simulink model "PUMA_PID_dis"  (Simulink 8.9)
settings: Solver=ode15s  StartTime=0  StopTime=5  MaxStep=0.02  RelTol=1e-3  EnableMultiTasking=on
undefined symbols (not defined in the file): sfunxyz
libraries: aerolibutil x17, simulink x7
(part 1 of 3)
settings Model: Creator=LAAAS3  LastModifiedBy=bmoh1
settings OptimizationCC: InitFltsAndDblsToZero=on
settings DebuggingCC: SaveWithParameterizedLinksMsg=none  SignalResolutionControl=TryResolveAllWithWarning  MaxConsecutiveZCsMsg=none  SolverPrmCheckMsg=warning  MultiTaskDSMMsg=warning  MultiTaskCondExecSysMsg=none  FcnCallInpInsideContextMsg=error  StateNameClashWarn=none
settings GRTTargetCC: TargetFcnLib=ansi_tfl_tmw.mat  GeneratePreprocessorConditionals=Use local settings

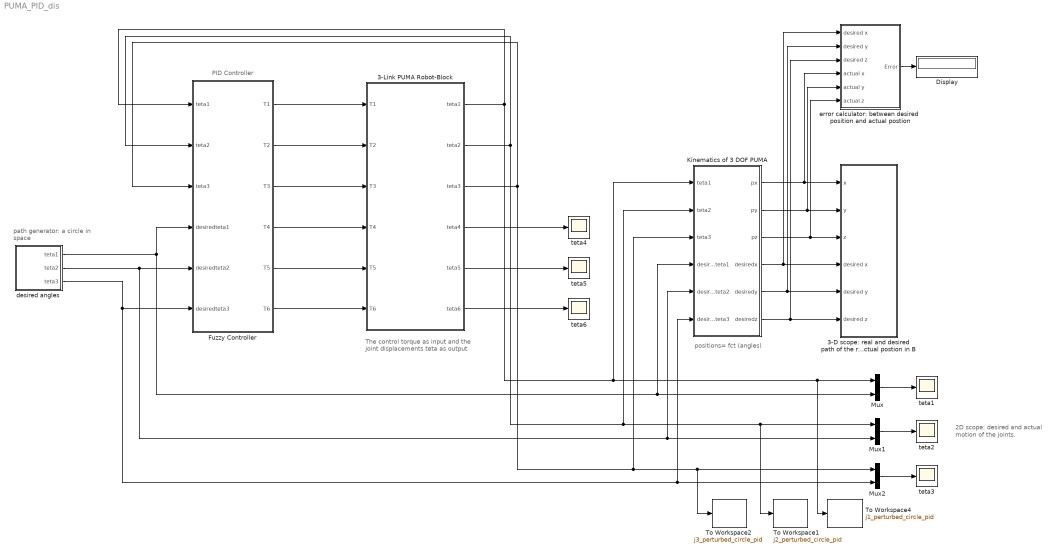
== system PUMA_PID_dis ==
  note: PID Controller
  note: 2D scope: desired and actual
      |          motion of the joints.
  note: The control torque as input and the
      | joint displacements teta as output
  note: path generator: a
      | circle in space
  note: positions= fct (angles)
  "3-D scope: real and desired path of the robot  desired position in G and actual postion in B " : Subsystem
  "3-Link PUMA Robot-Block " : Subsystem  mask{UIm1=0, UIm2=0, UIm3=0, UIm4=0, UIm5=0, UIm6=0, UI1=0, UI2=0, UI3=0, UI4=0, UI5=0, UI6=0, UI7=0, UI8=0, UI9=0, UI10=0, UI11=0, UI12=0, UI13=0, UI14=0, UI15=0, UI16=0, UI17=0, UI18=0, UI19=0, UI20=0, UI21=0, UI22=0, UI23=0, UG1=0, UG2=0, UG3=0, UG4=0, UG5=0}
      mask prompts: UIm1 "UIm1 +-0.27"; UIm2 "UIm2 +-0.54"; UIm3 "UIm3 +-0.093"; UIm4 "UIm4 +-0.016"; UIm5 "UIm5 +-0.014"; UIm6 "UIm6 +-0.016"; UI1 "UI1 +-0.05"; UI2 "UI2 +-0.07"; UI3 "UI3 +-0.05"; UI4 "UI4 +-0.02"; UI5 "UI5 +-0.031"; UI6 "UI6 +-0.016"; UI7 "UI7 +-0.029"; UI8 "UI8 +-0.014"; UI9 "UI9 +-0.012"; UI10 "UI10 +-0.0022"; UI11 "UI11 +-0.007"; UI12 "UI12 +-0.0011"; UI13 "UI13 +-0.0009"; UI14 "UI14 +-0.00007"; UI15 "UI15 +-0.0003"; UI16 "UI16 +-0.0003"; UI17 "UI17 +-0.0003"; UI18 "UI18 +-0.00013"; UI19 "UI19 +-0.0014"; UI20 "UI20 +-0.0008"; UI21 "UI21 +-0.0006"; UI22 "UI22 +-0.000015"; UI23 "UI23 +-0.00002"; UG1 "UG1 +-0.5"; UG2 "UG2 +-0.2"; UG3 "UG3 +-0.5"; UG4 "UG4 +-0.025"; UG5 "UG5 +-0.0056"
  Display : Display
  Fuzzy Controller : Subsystem
  Kinematics of 3 DOF PUMA : MATLAB Function  TreatAsAtomicUnit=on
  Mux : Mux  Inputs=2
  Mux1 : Mux  Inputs=2
  Mux2 : Mux  Inputs=2
  To Workspace1 : ToWorkspace  VariableName=j2_perturbed_circle_pid  SaveFormat=Timeseries  SampleTime=-1
      settings: Save2DSignal=2-D array (concatenate along first dimension)
  To Workspace2 : ToWorkspace  VariableName=j3_perturbed_circle_pid  SaveFormat=Timeseries  SampleTime=-1
      settings: Save2DSignal=2-D array (concatenate along first dimension)
  To Workspace4 : ToWorkspace  VariableName=j1_perturbed_circle_pid  SaveFormat=Timeseries  SampleTime=-1
      settings: Save2DSignal=2-D array (concatenate along first dimension)
  "desired angles  " : Subsystem
  error calculator: between desired  position and actual postion : Subsystem
  teta{1..6} (6 alike) : Scope
  wires:
  "3-Link PUMA Robot-Block "/3(teta3) -> To Workspace2/1, Mux2/1, Kinematics of 3 DOF PUMA/3(teta3), Fuzzy Controller/3(teta3)
  "3-Link PUMA Robot-Block "/4(teta4) -> teta4/1
  "3-Link PUMA Robot-Block "/5(teta5) -> teta5/1
  "3-Link PUMA Robot-Block "/6(teta6) -> teta6/1
  "desired angles  "/1(teta1) -> Mux/2, Kinematics of 3 DOF PUMA/4(desiredteta1), Fuzzy Controller/4(desiredteta1)
  "desired angles  "/2(teta2) -> Mux1/2, Kinematics of 3 DOF PUMA/5(desiredteta2), Fuzzy Controller/5(desiredteta2)
  "desired angles  "/3(teta3) -> Mux2/2, Kinematics of 3 DOF PUMA/6(desiredteta3), Fuzzy Controller/6(desiredteta3)
  error calculator: between desired  position and actual postion/1(Error) -> Display/1
  Kinematics of 3 DOF PUMA/1(px) -> "3-D scope: real and desired path of the robot  desired position in G and actual postion in B "/1(x), error calculator: between desired  position and actual postion/4(actual x)
  Kinematics of 3 DOF PUMA/2(py) -> "3-D scope: real and desired path of the robot  desired position in G and actual postion in B "/2(y), error calculator: between desired  position and actual postion/5(actual y)
  Kinematics of 3 DOF PUMA/3(pz) -> "3-D scope: real and desired path of the robot  desired position in G and actual postion in B "/3(z), error calculator: between desired  position and actual postion/6(actual z)
  Kinematics of 3 DOF PUMA/4(desiredx) -> "3-D scope: real and desired path of the robot  desired position in G and actual postion in B "/4(desired x), error calculator: between desired  position and actual postion/1(desired x)
  Kinematics of 3 DOF PUMA/5(desiredy) -> "3-D scope: real and desired path of the robot  desired position in G and actual postion in B "/5(desired y), error calculator: between desired  position and actual postion/2(desired y)
  Kinematics of 3 DOF PUMA/6(desiredz) -> "3-D scope: real and desired path of the robot  desired position in G and actual postion in B "/6(desired z), error calculator: between desired  position and actual postion/3(desired z)
  Mux/1 -> teta1/1
  Mux1/1 -> teta2/1
  Mux2/1 -> teta3/1
  Fuzzy Controller/4(T4) -> "3-Link PUMA Robot-Block "/4(T4)
  Fuzzy Controller/5(T5) -> "3-Link PUMA Robot-Block "/5(T5)
  Fuzzy Controller/6(T6) -> "3-Link PUMA Robot-Block "/6(T6)
  Fuzzy Controller/1(T1) -> "3-Link PUMA Robot-Block "/1(T1)
  Fuzzy Controller/2(T2) -> "3-Link PUMA Robot-Block "/2(T2)
  Fuzzy Controller/3(T3) -> "3-Link PUMA Robot-Block "/3(T3)
  "3-Link PUMA Robot-Block "/2(teta2) -> To Workspace1/1, Mux1/1, Kinematics of 3 DOF PUMA/2(teta2), Fuzzy Controller/2(teta2)
  "3-Link PUMA Robot-Block "/1(teta1) -> To Workspace4/1, Mux/1, Kinematics of 3 DOF PUMA/1(teta1), Fuzzy Controller/1(teta1)

== system PUMA_PID_dis/3-D scope: real and desired path of the robot  desired position in G and actual postion in B  ==
  x : Inport
  y : Inport  Port=2
  z : Inport  Port=3
  desired x : Inport  Port=4
  desired y : Inport  Port=5
  desired z : Inport  Port=6
  Demux : Demux  Outputs=[2 2 2]
  Mux : Mux  Inputs=3
  Mux1 : Mux  Inputs=3
  Mux3 : Mux  Inputs=2
  To Workspace1 : ToWorkspace  VariableName=xyz_pert_circle_pid  SaveFormat=Timeseries  SampleTime=-1
      settings: Save2DSignal=2-D array (concatenate along first dimension)
  Transpose : Selector  InputPortWidth=3*2  IndexOptions=Index vector (dialog)  Indices=reshape(reshape(1:3*2,3,2)',3*2,1)  OutputSizes=1
  XYZ Graph : Subsystem  LoadFcn=sfunxyz([],[],[],'LoadBlock')  StartFcn=sfunxyz([],[],[],'Start')  StopFcn=sfunxyz([],[],[],'Stop')  mask(XYZ multiscope){np=2, xlim=[-1 1], ylim=[-1 1], zlim=[-1 1], cp=[3 2 1], gd=on, st=0.1}
      mask prompts: np "Number of lines"; xlim "[xmin xmax]"; ylim "[ymin ymax]"; zlim "[zmin zmax]"; cp "Camera position (use [0 0 1] for 2D XY view)"; gd "Grid"; st "Sample time:"
      mask help:
      | Multidimensional XYZ scope using MATLAB graph window.
      |    X,Y,Z coordinates are respectively the first,second, and third input.
      |    Enter the number of lines, the XYZ ranges, the camera position,
      |    and the sampling time, as mask parameters.
      settings: CopyFcn=sfunxyz([],[],[],'CopyBlock')  DeleteFcn=sfunxyz([],[],[],'DeleteBlock')  NameChangeFcn=sfunxyz([],[],[],'NameChange')
      mask Help:
      | This block can be used to explore limit cycles.
      |    Look at the m-file sfunxyz.m to see how it works.
      mask Display: plot([.05 .95 .95 .05 .05],[.45 .45 .95 .95 .45], 0.5+cos(0:0.1:2*pi)*0.3,0.7+sin(0:0.1:2*pi)*0.2)
  wires:
  Mux1/1 -> Mux3/2  "Line2 XYZ"
  Mux3/1 -> Transpose/1
  Transpose/1 -> Demux/1
  Demux/1 -> XYZ Graph/1(x)  "X Coordinates"
  Demux/2 -> XYZ Graph/2(y)  "Y Coordinates"
  Demux/3 -> XYZ Graph/3(z)  "Z Coordinates"
  x/1 -> Mux/1
  y/1 -> Mux/2
  z/1 -> Mux/3
  Mux/1 -> To Workspace1/1, Mux3/1  "Line1 XYZ"
  desired x/1 -> Mux1/1
  desired y/1 -> Mux1/2
  desired z/1 -> Mux1/3

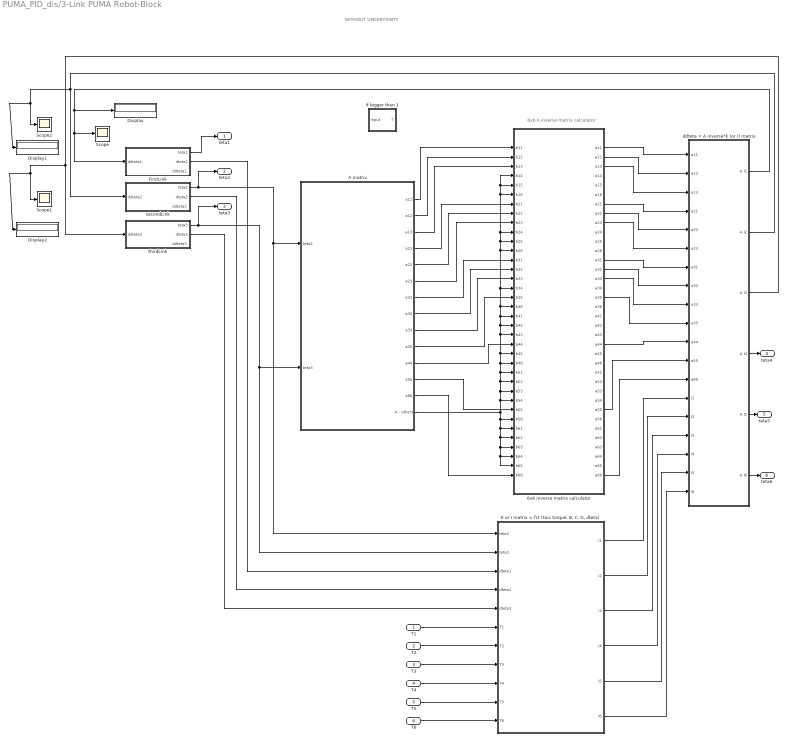
== system PUMA_PID_dis/3-Link PUMA Robot-Block  ==
  note: 6x6 A inverse matrix calculator
  note: WITHOUT UNCERTAINTY
  T1 : Inport
  T2 : Inport  Port=2
  T3 : Inport  Port=3
  T4 : Inport  Port=4
  T5 : Inport  Port=5
  T6 : Inport  Port=6
  6x6 inverse matrix calculator : MATLAB Function  TreatAsAtomicUnit=on
  A matrix : Subsystem
  Display : Display
  Display1 : Display
  Display2 : Display
  FirstLink : Subsystem  mask(FirstLink){}
      mask help:
      | the first link of the robot. the input is the double derivative of teta1, the displacement of
      | the link.
      | the outputs are: teta1 the displacement of the first joint, dteta1 the velocity of the
      | first joint.
      | NOTE: the link is connected to a revolute joint.
      mask Help:
      | the first link of the robot. the input is the double derivative of teta1, the displacement of
      | the link.
      | the outputs are: teta1 the displacement of the first joint, dteta1 the velocity of the
      | first joint.
      | NOTE: the link is connected to a revolute joint.
  "K or I matrix = fct (tau: torque, B, C, G, dteta) " : Subsystem
  Scope : Scope
  Scope1 : Scope
  Scope2 : Scope
  "ddteta = A inverse*k (or I) matrix " : Subsystem
  if bigger than 1 : MATLAB Function  TreatAsAtomicUnit=on
  secondLink : Subsystem  mask(SecondLink){}
      mask help:
      | the first link of the robot. the input is the double derivative of teta1, the displacement of
      | the link.
      | the outputs are: teta1 the displacement of the second joint, dteta1 the velocity of the
      | second joint.
      | NOTE: the link is connected to a revolute joint.
      mask Help:
      | the secod link of the robot. the input is the double derivative of teta2, the displacement of
      | the link.
      | the outputs are: teta2 the displacement of the second joint, dteta2 the velocity of the
      | second joint.
      | NOTE: the link is connected to a revolute joint.
  thirdLink : Subsystem  mask(ThirdLink){}
      mask help:
      | the third link of the robot. the input is the double derivative of teta3, the displacement of
      | the link.
      | the outputs are: teta3 the displacement of the third joint, dteta3 the velocity of the
      | third joint.
      | NOTE: the link is connected to a revolute joint.
      mask Help:
      | the third link of the robot. the input is the double derivative of teta3, the displacement of
      | the link.
      | the outputs are: teta3 the displacement of the third joint, dteta3 the velocity of the
      | third joint.
      | NOTE: the link is connected to a revolute joint.
  teta1 : Outport
  teta2 : Outport  Port=2
  teta3 : Outport  Port=3
  teta4 : Outport  Port=4
  teta5 : Outport  Port=5
  teta6 : Outport  Port=6
  wires:
  A matrix/1(a11) -> 6x6 inverse matrix calculator/1(b11)
  A matrix/2(a12) -> 6x6 inverse matrix calculator/2(b12)
  A matrix/3(a13) -> 6x6 inverse matrix calculator/3(b13)
  A matrix/4(a21) -> 6x6 inverse matrix calculator/7(b21)
  A matrix/5(a22) -> 6x6 inverse matrix calculator/8(b22)
  A matrix/6(a23) -> 6x6 inverse matrix calculator/9(b23)
  A matrix/7(a31) -> 6x6 inverse matrix calculator/13(b31)
  A matrix/8(a32) -> 6x6 inverse matrix calculator/14(b32)
  A matrix/9(a33) -> 6x6 inverse matrix calculator/15(b33)
  A matrix/10(a35) -> 6x6 inverse matrix calculator/17(b35)
  A matrix/11(a44) -> 6x6 inverse matrix calculator/22(b44)
  A matrix/12(a55) -> 6x6 inverse matrix calculator/29(b55)
  A matrix/13(a66) -> 6x6 inverse matrix calculator/36(b66)
  A matrix/14(A - others) -> 6x6 inverse matrix calculator/30(b56), 6x6 inverse matrix calculator/35(b65), 6x6 inverse matrix calculator/34(b64), 6x6 inverse matrix calculator/33(b63), 6x6 inverse matrix calculator/32(b62), 6x6 inverse matrix calculator/31(b61), 6x6 inverse matrix calculator/28(b54), 6x6 inverse matrix calculator/27(b53), 6x6 inverse matrix calculator/26(b52), 6x6 inverse matrix calculator/25(b51), 6x6 inverse matrix calculator/24(b46), 6x6 inverse matrix calculator/23(b45), 6x6 inverse matrix calculator/21(b43), 6x6 inverse matrix calculator/20(b42), 6x6 inverse matrix calculator/19(b41), 6x6 inverse matrix calculator/18(b36), 6x6 inverse matrix calculator/16(b34), 6x6 inverse matrix calculator/12(b26), 6x6 inverse matrix calculator/11(b25), 6x6 inverse matrix calculator/10(b24), 6x6 inverse matrix calculator/6(b16), 6x6 inverse matrix calculator/4(b14), 6x6 inverse matrix calculator/5(b15)
  secondLink/1(teta2) -> "K or I matrix = fct (tau: torque, B, C, G, dteta) "/1(teta2), A matrix/1(teta2), teta2/1
  thirdLink/1(teta3) -> teta3/1, "K or I matrix = fct (tau: torque, B, C, G, dteta) "/2(teta3), A matrix/2(teta3)
  FirstLink/2(dteta1) -> "K or I matrix = fct (tau: torque, B, C, G, dteta) "/3(dteta1)
  secondLink/2(dteta2) -> "K or I matrix = fct (tau: torque, B, C, G, dteta) "/4(dteta2)
  thirdLink/2(dteta3) -> "K or I matrix = fct (tau: torque, B, C, G, dteta) "/5(dteta3)
  T1/1 -> "K or I matrix = fct (tau: torque, B, C, G, dteta) "/6(T1)
  T2/1 -> "K or I matrix = fct (tau: torque, B, C, G, dteta) "/7(T2)
  T3/1 -> "K or I matrix = fct (tau: torque, B, C, G, dteta) "/8(T3)
  T4/1 -> "K or I matrix = fct (tau: torque, B, C, G, dteta) "/9(T4)
  T5/1 -> "K or I matrix = fct (tau: torque, B, C, G, dteta) "/10(T5)
  T6/1 -> "K or I matrix = fct (tau: torque, B, C, G, dteta) "/11(T6)
  "ddteta = A inverse*k (or I) matrix "/1(A.I1) -> Display/1, Scope/1, FirstLink/1(ddteta1)
  FirstLink/1(teta1) -> teta1/1
  "ddteta = A inverse*k (or I) matrix "/4(A.I4) -> teta4/1
  "ddteta = A inverse*k (or I) matrix "/5(A.I5) -> teta5/1
  "ddteta = A inverse*k (or I) matrix "/6(A.I6) -> teta6/1
  "K or I matrix = fct (tau: torque, B, C, G, dteta) "/1(I1) -> "ddteta = A inverse*k (or I) matrix "/14(I1)
  "K or I matrix = fct (tau: torque, B, C, G, dteta) "/2(I2) -> "ddteta = A inverse*k (or I) matrix "/15(I2)
  "K or I matrix = fct (tau: torque, B, C, G, dteta) "/3(I3) -> "ddteta = A inverse*k (or I) matrix "/16(I3)
  6x6 inverse matrix calculator/1(a11) -> "ddteta = A inverse*k (or I) matrix "/1(a11)
  6x6 inverse matrix calculator/2(a12) -> "ddteta = A inverse*k (or I) matrix "/2(a12)
  6x6 inverse matrix calculator/3(a13) -> "ddteta = A inverse*k (or I) matrix "/3(a13)
  6x6 inverse matrix calculator/7(a21) -> "ddteta = A inverse*k (or I) matrix "/4(a21)
  6x6 inverse matrix calculator/8(a22) -> "ddteta = A inverse*k (or I) matrix "/5(a22)
  6x6 inverse matrix calculator/9(a23) -> "ddteta = A inverse*k (or I) matrix "/6(a23)
  6x6 inverse matrix calculator/13(a31) -> "ddteta = A inverse*k (or I) matrix "/7(a31)
  6x6 inverse matrix calculator/14(a32) -> "ddteta = A inverse*k (or I) matrix "/8(a32)
  6x6 inverse matrix calculator/15(a33) -> "ddteta = A inverse*k (or I) matrix "/9(a33)
  6x6 inverse matrix calculator/17(a35) -> "ddteta = A inverse*k (or I) matrix "/10(a35)
  6x6 inverse matrix calculator/22(a44) -> "ddteta = A inverse*k (or I) matrix "/11(a44)
  6x6 inverse matrix calculator/29(a55) -> "ddteta = A inverse*k (or I) matrix "/12(a55)
  6x6 inverse matrix calculator/36(a66) -> "ddteta = A inverse*k (or I) matrix "/13(a66)
  "K or I matrix = fct (tau: torque, B, C, G, dteta) "/4(I4) -> "ddteta = A inverse*k (or I) matrix "/17(I4)
  "K or I matrix = fct (tau: torque, B, C, G, dteta) "/5(I5) -> "ddteta = A inverse*k (or I) matrix "/18(I5)
  "K or I matrix = fct (tau: torque, B, C, G, dteta) "/6(I6) -> "ddteta = A inverse*k (or I) matrix "/19(I6)
  "ddteta = A inverse*k (or I) matrix "/3(A.I3) -> Display2/1, Scope1/1, thirdLink/1(ddteta3)
  "ddteta = A inverse*k (or I) matrix "/2(A.I2) -> Display1/1, Scope2/1, secondLink/1(ddteta2)

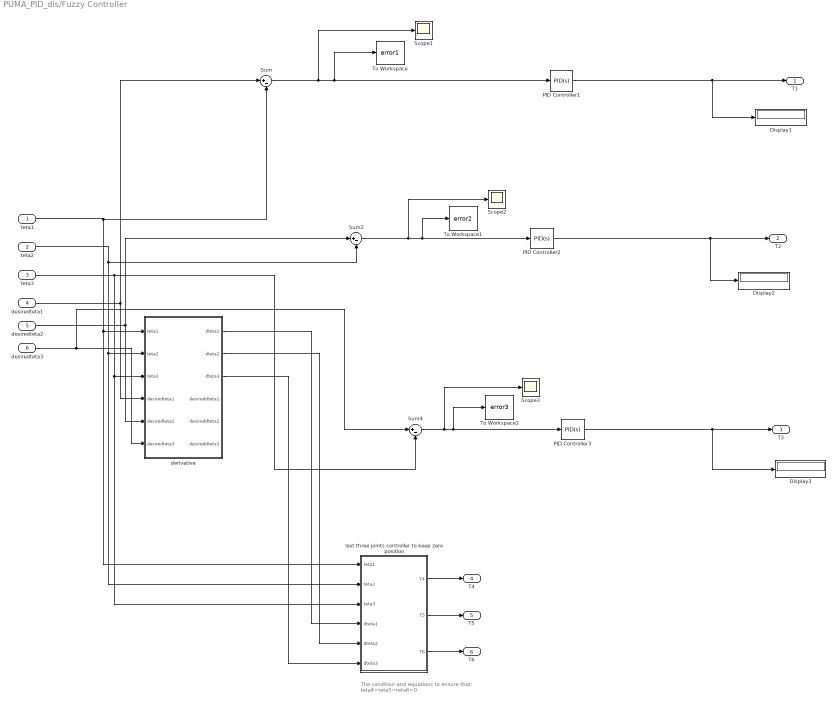
== system PUMA_PID_dis/Fuzzy Controller ==
  note: The condition and equations to ensure that:
      |                    teta4=teta5=teta6=0
  teta1 : Inport
  teta2 : Inport  Port=2
  teta3 : Inport  Port=3
  desiredteta1 : Inport  Port=4
  desiredteta2 : Inport  Port=5
  desiredteta3 : Inport  Port=6
  Display1 : Display
  Display2 : Display
  Display3 : Display
  PID Controller1 : simulink/Continuous/PID Controller  Controller=PID  TimeDomain=Continuous-time  SampleTime=-1  IntegratorMethod=Forward Euler  FilterMethod=Forward Euler  Form=Parallel  UseFilter=on  ControllerParametersSource=internal  P=100  I=1  D=60  N=38.4128689358779  InitialConditionSource=internal  InitialConditionForIntegrator=0  InitialConditionForFilter=0  ExternalReset=none  LimitOutput=off  UpperSaturationLimit=inf  LowerSaturationLimit=-inf  LinearizeAsGain=on  AntiWindupMode=none  Kb=1  TrackingMode=off  Kt=1  PParamMin=[]  PParamMax=[]  IParamMin=[]  IParamMax=[]  DParamMin=[]  DParamMax=[]  NParamMin=[]  NParamMax=[]  KbParamMin=[]  KbParamMax=[]  KtParamMin=[]  KtParamMax=[]  POutMin=[]  POutMax=[]  IOutMin=[]  IOutMax=[]  DOutMin=[]  DOutMax=[]  NOutMin=[]  NOutMax=[]  KbOutMin=[]  KbOutMax=[]  KtOutMin=[]  KtOutMax=[]  IntegratorOutMin=[]  IntegratorOutMax=[]  FilterOutMin=[]  FilterOutMax=[]  SumOutMin=[]  SumOutMax=[]  SumI1OutMin=[]  SumI1OutMax=[]  SumI2OutMin=[]  SumI2OutMax=[]  SumI3OutMin=[]  SumI3OutMax=[]  SumDOutMin=[]  SumDOutMax=[]  SaturationOutMin=[]  SaturationOutMax=[]  IntegratorContinuousStateAttributes=''  IntegratorStateMustResolveToSignalObject=off  IntegratorRTWStateStorageClass=Auto  FilterContinuousStateAttributes=''  FilterStateMustResolveToSignalObject=off  FilterRTWStateStorageClass=Auto  DifferentiatorICPrevScaledInput=0  DifferentiatorOutMin=[]  DifferentiatorOutMax=[]  InitialConditionSetting=State (most efficient)
  PID Controller2 : simulink/Continuous/PID Controller  Controller=PID  TimeDomain=Continuous-time  SampleTime=-1  IntegratorMethod=Forward Euler  FilterMethod=Forward Euler  Form=Parallel  UseFilter=on  ControllerParametersSource=internal  P=259.447618274315  I=64.6556993070995  D=70.4723983176902  N=17.7020176521094  InitialConditionSource=internal  InitialConditionForIntegrator=0  InitialConditionForFilter=0  ExternalReset=none  LimitOutput=off  UpperSaturationLimit=inf  LowerSaturationLimit=-inf  LinearizeAsGain=on  AntiWindupMode=none  Kb=1  TrackingMode=off  Kt=1  PParamMin=[]  PParamMax=[]  IParamMin=[]  IParamMax=[]  DParamMin=[]  DParamMax=[]  NParamMin=[]  NParamMax=[]  KbParamMin=[]  KbParamMax=[]  KtParamMin=[]  KtParamMax=[]  POutMin=[]  POutMax=[]  IOutMin=[]  IOutMax=[]  DOutMin=[]  DOutMax=[]  NOutMin=[]  NOutMax=[]  KbOutMin=[]  KbOutMax=[]  KtOutMin=[]  KtOutMax=[]  IntegratorOutMin=[]  IntegratorOutMax=[]  FilterOutMin=[]  FilterOutMax=[]  SumOutMin=[]  SumOutMax=[]  SumI1OutMin=[]  SumI1OutMax=[]  SumI2OutMin=[]  SumI2OutMax=[]  SumI3OutMin=[]  SumI3OutMax=[]  SumDOutMin=[]  SumDOutMax=[]  SaturationOutMin=[]  SaturationOutMax=[]  IntegratorContinuousStateAttributes=''  IntegratorStateMustResolveToSignalObject=off  IntegratorRTWStateStorageClass=Auto  FilterContinuousStateAttributes=''  FilterStateMustResolveToSignalObject=off  FilterRTWStateStorageClass=Auto  DifferentiatorICPrevScaledInput=0  DifferentiatorOutMin=[]  DifferentiatorOutMax=[]  InitialConditionSetting=State (most efficient)
  PID Controller3 : simulink/Continuous/PID Controller  Controller=PID  TimeDomain=Continuous-time  SampleTime=-1  IntegratorMethod=Forward Euler  FilterMethod=Forward Euler  Form=Parallel  UseFilter=on  ControllerParametersSource=internal  P=298.294353009705  I=370.312527265234  D=35  N=2913.028427628  InitialConditionSource=internal  InitialConditionForIntegrator=0  InitialConditionForFilter=0  ExternalReset=none  LimitOutput=off  UpperSaturationLimit=inf  LowerSaturationLimit=-inf  LinearizeAsGain=on  AntiWindupMode=none  Kb=1  TrackingMode=off  Kt=1  PParamMin=[]  PParamMax=[]  IParamMin=[]  IParamMax=[]  DParamMin=[]  DParamMax=[]  NParamMin=[]  NParamMax=[]  KbParamMin=[]  KbParamMax=[]  KtParamMin=[]  KtParamMax=[]  POutMin=[]  POutMax=[]  IOutMin=[]  IOutMax=[]  DOutMin=[]  DOutMax=[]  NOutMin=[]  NOutMax=[]  KbOutMin=[]  KbOutMax=[]  KtOutMin=[]  KtOutMax=[]  IntegratorOutMin=[]  IntegratorOutMax=[]  FilterOutMin=[]  FilterOutMax=[]  SumOutMin=[]  SumOutMax=[]  SumI1OutMin=[]  SumI1OutMax=[]  SumI2OutMin=[]  SumI2OutMax=[]  SumI3OutMin=[]  SumI3OutMax=[]  SumDOutMin=[]  SumDOutMax=[]  SaturationOutMin=[]  SaturationOutMax=[]  IntegratorContinuousStateAttributes=''  IntegratorStateMustResolveToSignalObject=off  IntegratorRTWStateStorageClass=Auto  FilterContinuousStateAttributes=''  FilterStateMustResolveToSignalObject=off  FilterRTWStateStorageClass=Auto  DifferentiatorICPrevScaledInput=0  DifferentiatorOutMin=[]  DifferentiatorOutMax=[]  InitialConditionSetting=State (most efficient)
  Scope1 : Scope
  Scope2 : Scope
  Scope3 : Scope
  Sum : Sum  Inputs=|+-
  Sum2 : Sum  Inputs=|+-
  Sum4 : Sum  Inputs=|+-
  To Workspace : ToWorkspace  VariableName=error1  SampleTime=-1
      settings: Save2DSignal=2-D array (concatenate along first dimension)
  To Workspace1 : ToWorkspace  VariableName=error2  SampleTime=-1
      settings: Save2DSignal=2-D array (concatenate along first dimension)
  To Workspace2 : ToWorkspace  VariableName=error3  SampleTime=-1
      settings: Save2DSignal=2-D array (concatenate along first dimension)
  derivative : Subsystem
  last three joints controller to keep zero position : MATLAB Function  TreatAsAtomicUnit=on
  T1 : Outport
  T2 : Outport  Port=2
  T3 : Outport  Port=3
  T4 : Outport  Port=4
  T5 : Outport  Port=5
  T6 : Outport  Port=6
  wires:
  derivative/1(dteta1) -> last three joints controller to keep zero position/4(dteta1)
  derivative/2(dteta2) -> last three joints controller to keep zero position/5(dteta2)
  derivative/3(dteta3) -> last three joints controller to keep zero position/6(dteta3)
  teta1/1 -> Sum/2, derivative/1(teta1), last three joints controller to keep zero position/1(teta1)
  teta2/1 -> Sum2/2, derivative/2(teta2), last three joints controller to keep zero position/2(teta2)
  teta3/1 -> Sum4/2, derivative/3(teta3), last three joints controller to keep zero position/3(teta3)
  desiredteta1/1 -> Sum/1, derivative/4(desiredteta1)
  desiredteta2/1 -> Sum2/1, derivative/5(desiredteta2)
  desiredteta3/1 -> Sum4/1, derivative/6(desiredteta3)
  last three joints controller to keep zero position/1(T4) -> T4/1
  last three joints controller to keep zero position/2(T5) -> T5/1
  last three joints controller to keep zero position/3(T6) -> T6/1
  Sum/1 -> Scope1/1, To Workspace/1, PID Controller1/1
  Sum2/1 -> Scope2/1, To Workspace1/1, PID Controller2/1
  PID Controller2/1 -> Display2/1, T2/1
  Sum4/1 -> Scope3/1, To Workspace2/1, PID Controller3/1
  PID Controller1/1 -> Display1/1, T1/1
  PID Controller3/1 -> Display3/1, T3/1

== system PUMA_PID_dis/desired angles   ==
  Add1 : Sum
  Add2 : Sum
  Constant : Constant  Value=0
  Ramp2 : simulink/Sources/Ramp  slope=-2  start=3.33  X0=0
  Ramp4 : simulink/Sources/Ramp  slope=2  start=0  X0=0
  Ramp5 : simulink/Sources/Ramp  slope=2  start=3.33  X0=0
  Ramp6 : simulink/Sources/Ramp  slope=-2  start=0  X0=0
  Scope : Scope
  Scope1 : Scope
  Scope2 : Scope
  teta1 : Outport
  teta2 : Outport  Port=2
  teta3 : Outport  Port=3
  wires:
  Ramp4/1 -> Add1/1
  Ramp2/1 -> Add1/2
  Ramp6/1 -> Add2/1
  Ramp5/1 -> Add2/2
  Constant/1 -> Scope/1, teta1/1
  Add1/1 -> Scope1/1, teta2/1
  Add2/1 -> Scope2/1, teta3/1

== system PUMA_PID_dis/error calculator: between desired  position and actual postion ==
  note: Error = sqrt ((acyual x - desired x)^2 + (acyual y - desired y)^2 + (acyual z - desired z)^2)
  desired x : Inport
  desired y : Inport  Port=2
  desired z : Inport  Port=3
  actual x : Inport  Port=4
  actual y : Inport  Port=5
  actual z : Inport  Port=6
  Add : Sum  Inputs=-+
  Add1 : Sum  Inputs=-+
  Add2 : Sum  Inputs=-+
  Add3 : Sum  Inputs=+++
  Scope Total RMSE : Scope
  To Workspace : ToWorkspace  VariableName=error  SampleTime=-1
      settings: Save2DSignal=2-D array (concatenate along first dimension)
  To Workspace1 : ToWorkspace  VariableName=error4  SampleTime=-1
      settings: Save2DSignal=2-D array (concatenate along first dimension)
  To Workspace2 : ToWorkspace  VariableName=error5  SampleTime=-1
      settings: Save2DSignal=2-D array (concatenate along first dimension)
  To Workspace3 : ToWorkspace  VariableName=error6  SampleTime=-1
      settings: Save2DSignal=2-D array (concatenate along first dimension)
  Error : Outport
  wires:
  desired x/1 -> Add/1
  actual x/1 -> Add/2
  desired y/1 -> Add1/1
  actual y/1 -> Add1/2
  desired z/1 -> Add2/1
  actual z/1 -> Add2/2
  Add1/1 -> To Workspace2/1, Add3/2
  Add/1 -> To Workspace1/1, Add3/1
  Add3/1 -> Scope Total RMSE/1, To Workspace/1, Error/1
  Add2/1 -> To Workspace3/1, Add3/3

== system PUMA_PID_dis/3-D scope: real and desired path of the robot  desired position in G and actual postion in B /XYZ Graph ==
  x : Inport
  y : Inport  Port=2
  z : Inport  Port=3
  Mux : Mux  Inputs=[np np np]
  sfunxy : S-Function  FunctionName=sfunxyz  Parameters=[xlim ylim zlim],st,np,cp,gd  SFunctionDeploymentMode=off  EnableBusSupport=off
  wires:
  z/1 -> Mux/3
  y/1 -> Mux/2
  x/1 -> Mux/1
  Mux/1 -> sfunxy/1

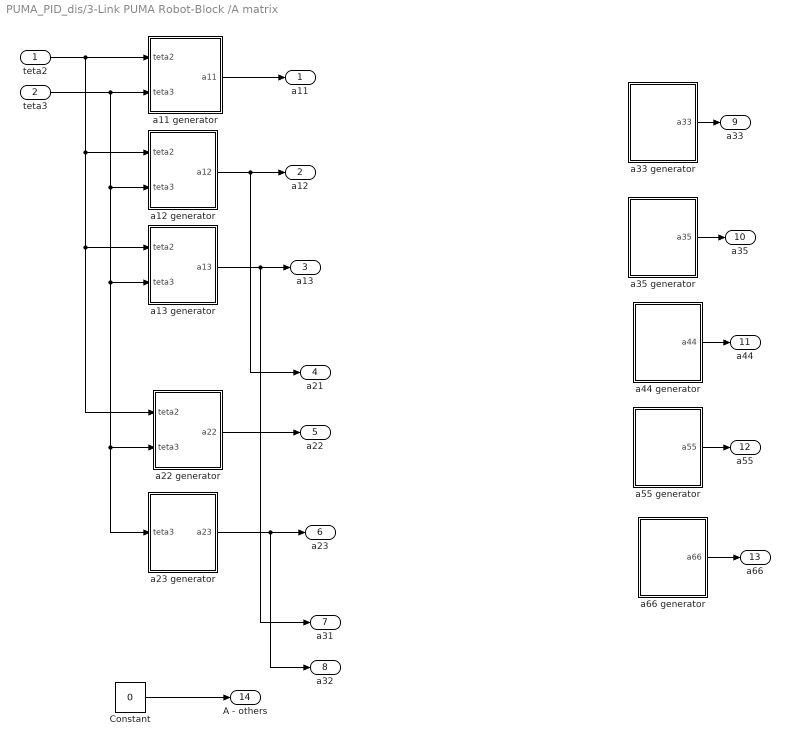
== system PUMA_PID_dis/3-Link PUMA Robot-Block /A matrix ==
  teta2 : Inport
  teta3 : Inport  Port=2
  Constant : Constant  Value=0
  a11 generator : Subsystem
  a12 generator : Subsystem
  a13 generator : Subsystem
  a22 generator : Subsystem
  a23 generator : Subsystem
  a33 generator : Subsystem
  a35 generator : Subsystem
  a44 generator : Subsystem
  a55 generator : Subsystem
  a66 generator : Subsystem
  a11 : Outport
  a12 : Outport  Port=2
  a13 : Outport  Port=3
  a21 : Outport  Port=4
  a22 : Outport  Port=5
  a23 : Outport  Port=6
  a31 : Outport  Port=7
  a32 : Outport  Port=8
  a33 : Outport  Port=9
  a35 : Outport  Port=10
  a44 : Outport  Port=11
  a55 : Outport  Port=12
  a66 : Outport  Port=13
  A - others : Outport  Port=14
  wires:
  a11 generator/1(a11) -> a11/1
  a12 generator/1(a12) -> a12/1, a21/1
  a13 generator/1(a13) -> a13/1, a31/1
  Constant/1 -> A - others/1
  a22 generator/1(a22) -> a22/1
  a23 generator/1(a23) -> a23/1, a32/1
  a33 generator/1(a33) -> a33/1
  a35 generator/1(a35) -> a35/1
  a44 generator/1(a44) -> a44/1
  a55 generator/1(a55) -> a55/1
  a66 generator/1(a66) -> a66/1
  teta2/1 -> a22 generator/1(teta2), a13 generator/1(teta2), a12 generator/1(teta2), a11 generator/1(teta2)
  teta3/1 -> a23 generator/1(teta3), a22 generator/2(teta3), a13 generator/2(teta3), a12 generator/2(teta3), a11 generator/2(teta3)

== system PUMA_PID_dis/3-Link PUMA Robot-Block /FirstLink ==
  ddteta1 : Inport
  Integrator : Integrator  LimitOutput=on  UpperSaturationLimit=10  LowerSaturationLimit=-10
  Integrator1 : Integrator  LimitOutput=on  UpperSaturationLimit=10  LowerSaturationLimit=-10
  Scope : Scope
  teta1 : Outport
  dteta1 : Outport  Port=2
  ddteta1. : Outport  Port=3
  wires:
  ddteta1/1 -> Scope/1, Integrator/1, ddteta1./1
  Integrator/1 -> Integrator1/1, dteta1/1
  Integrator1/1 -> teta1/1

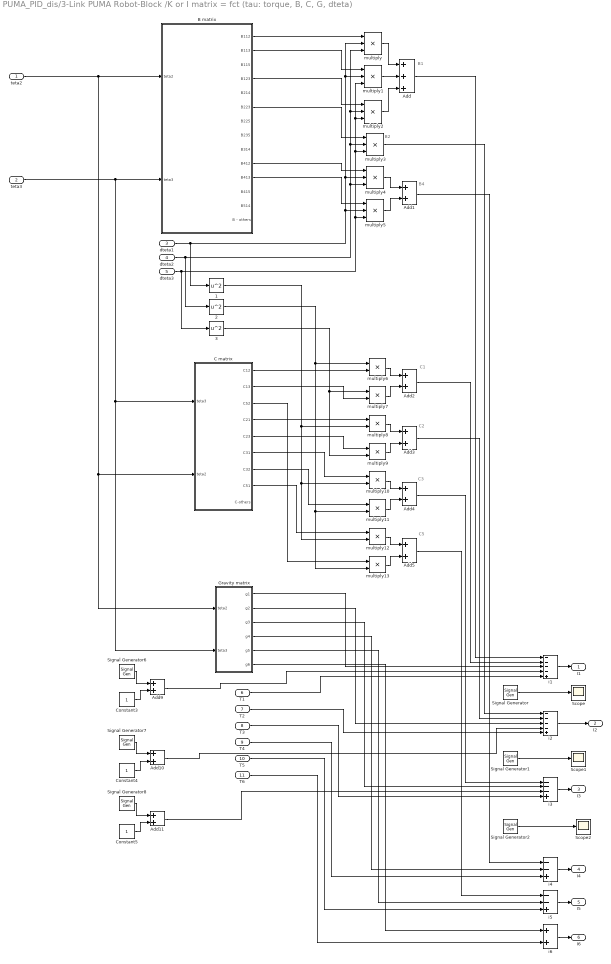
== system PUMA_PID_dis/3-Link PUMA Robot-Block /K or I matrix = fct (tau: torque, B, C, G, dteta)  ==
  note: B1
  note: B2
  note: B4
  note: C1
  note: C2
  note: C3
  note: C5
  teta2 : Inport
  teta3 : Inport  Port=2
  dteta1 : Inport  Port=3
  dteta2 : Inport  Port=4
  dteta3 : Inport  Port=5
  T1 : Inport  Port=6
  T2 : Inport  Port=7
  T3 : Inport  Port=8
  T4 : Inport  Port=9
  T5 : Inport  Port=10
  T6 : Inport  Port=11
  1 : Math  Operator=square  SaturateOnIntegerOverflow=on
  2 : Math  Operator=square  SaturateOnIntegerOverflow=on
  3 : Math  Operator=square  SaturateOnIntegerOverflow=on
  Add : Sum  Inputs=+++
  Add{1..5,9..11} (8 alike) : Sum
  B matrix : Subsystem
  C matrix : Subsystem
  Constant3 : Constant
  Constant4 : Constant
  Constant5 : Constant
  Gravity matrix : Subsystem
  Scope : Scope
  Scope1 : Scope
  Scope2 : Scope
  Signal Generator : SignalGenerator  Frequency=3.18
  Signal Generator1 : SignalGenerator  Amplitude=0.05  Frequency=3.18
  Signal Generator2 : SignalGenerator  Amplitude=0.1  Frequency=3.18
  Signal Generator6 : SignalGenerator  Frequency=3.18
  Signal Generator7 : SignalGenerator  Amplitude=0.05  Frequency=3.18
  Signal Generator8 : SignalGenerator  Amplitude=0.05  Frequency=3.18
  i1 : Sum  Inputs=----+
  i2 : Sum  Inputs=----+
  i3 : Sum  Inputs=---+
  i4 : Sum  Inputs=--+
  i5 : Sum  Inputs=--+
  i6 : Sum
  multiply{,1..5} (6 alike) : Product  Inputs=***
  multiply{6..13} (8 alike) : Product  Inputs=**
  I1 : Outport
  I2 : Outport  Port=2
  I3 : Outport  Port=3
  I4 : Outport  Port=4
  I5 : Outport  Port=5
  I6 : Outport  Port=6
  wires:
  teta2/1 -> Gravity matrix/1(teta2), C matrix/2(teta2), B matrix/1(teta2)
  teta3/1 -> Gravity matrix/2(teta3), C matrix/1(teta3), B matrix/2(teta3)
  dteta3/1 -> multiply5/3, multiply3/3, multiply2/3, multiply1/3, 3/1
  dteta2/1 -> multiply4/3, multiply3/2, multiply2/2, multiply/3, 2/1
  dteta1/1 -> multiply5/2, multiply4/2, multiply1/2, multiply/2, 1/1
  B matrix/1(B112) -> multiply/1
  B matrix/2(B113) -> multiply1/1
  B matrix/4(B123) -> multiply2/1
  multiply/1 -> Add/1
  multiply1/1 -> Add/2
  multiply2/1 -> Add/3
  B matrix/6(B223) -> multiply3/1
  B matrix/10(B412) -> multiply4/1
  B matrix/11(B413) -> multiply5/1
  multiply4/1 -> Add1/1
  multiply5/1 -> Add1/2
  2/1 -> multiply6/1, multiply11/2, multiply13/2
  C matrix/1(C12) -> multiply6/2
  3/1 -> multiply7/1, multiply9/2
  C matrix/2(C13) -> multiply7/2
  multiply6/1 -> Add2/1
  multiply7/1 -> Add2/2
  multiply8/1 -> Add3/1
  multiply9/1 -> Add3/2
  C matrix/4(C21) -> multiply8/1
  C matrix/5(C23) -> multiply9/1
  1/1 -> multiply8/2, multiply10/2, multiply12/2
  multiply10/1 -> Add4/1
  multiply11/1 -> Add4/2
  C matrix/6(C31) -> multiply10/1
  C matrix/7(C32) -> multiply11/1
  multiply12/1 -> Add5/1
  multiply13/1 -> Add5/2
  C matrix/8(C51) -> multiply12/1
  C matrix/3(C52) -> multiply13/1
  T1/1 -> i1/5
  Gravity matrix/1(g1) -> i1/3
  Add2/1 -> i1/2
  Add/1 -> i1/1
  T2/1 -> i2/5
  Gravity matrix/2(g2) -> i2/3
  Add3/1 -> i2/2
  multiply3/1 -> i2/1
  T3/1 -> i3/4
  Gravity matrix/3(g3) -> i3/2
  Add4/1 -> i3/1
  T4/1 -> i4/3
  Gravity matrix/4(g4) -> i4/2
  Add1/1 -> i4/1
  T5/1 -> i5/3
  Gravity matrix/5(g5) -> i5/2
  Add5/1 -> i5/1
  i1/1 -> I1/1
  i2/1 -> I2/1
  i3/1 -> I3/1
  i4/1 -> I4/1
  i5/1 -> I5/1
  i6/1 -> I6/1
  Gravity matrix/6(g6) -> i6/1
  T6/1 -> i6/2
  Signal Generator/1 -> Scope/1
  Signal Generator1/1 -> Scope1/1
  Signal Generator2/1 -> Scope2/1
  Constant3/1 -> Add9/2
  Signal Generator6/1 -> Add9/1
  Constant4/1 -> Add10/2
  Signal Generator7/1 -> Add10/1
  Constant5/1 -> Add11/2
  Signal Generator8/1 -> Add11/1
  Add9/1 -> i1/4
  Add10/1 -> i2/4
  Add11/1 -> i3/3

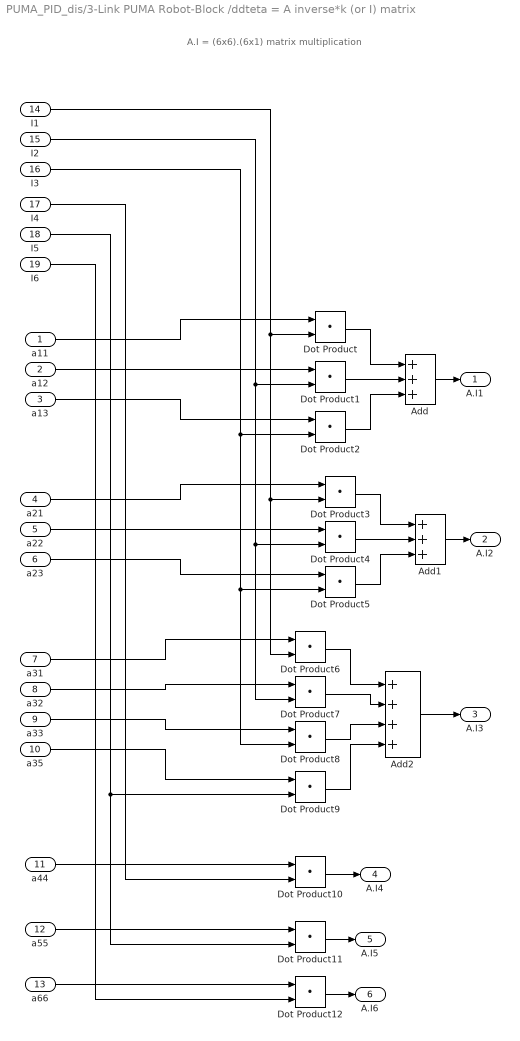
== system PUMA_PID_dis/3-Link PUMA Robot-Block /ddteta = A inverse*k (or I) matrix  ==
  note: A.I = (6x6).(6x1) matrix multiplication
  a11 : Inport
  a12 : Inport  Port=2
  a13 : Inport  Port=3
  a21 : Inport  Port=4
  a22 : Inport  Port=5
  a23 : Inport  Port=6
  a31 : Inport  Port=7
  a32 : Inport  Port=8
  a33 : Inport  Port=9
  a35 : Inport  Port=10
  a44 : Inport  Port=11
  a55 : Inport  Port=12
  a66 : Inport  Port=13
  I1 : Inport  Port=14
  I2 : Inport  Port=15
  I3 : Inport  Port=16
  I4 : Inport  Port=17
  I5 : Inport  Port=18
  I6 : Inport  Port=19
  Add : Sum  Inputs=+++
  Add1 : Sum  Inputs=+++
  Add2 : Sum  Inputs=++++
  Dot Product{,1..12} (13 alike) : DotProduct  InputSameDT=on  OutDataTypeStr=Inherit: Inherit via internal rule
  A.I1 : Outport
  A.I2 : Outport  Port=2
  A.I3 : Outport  Port=3
  A.I4 : Outport  Port=4
  A.I5 : Outport  Port=5
  A.I6 : Outport  Port=6
  wires:
  Dot Product/1 -> Add/1
  Dot Product1/1 -> Add/2
  Dot Product2/1 -> Add/3
  a11/1 -> Dot Product/1
  a12/1 -> Dot Product1/1
  a13/1 -> Dot Product2/1
  Dot Product3/1 -> Add1/1
  Dot Product4/1 -> Add1/2
  Dot Product5/1 -> Add1/3
  a21/1 -> Dot Product3/1
  a22/1 -> Dot Product4/1
  a23/1 -> Dot Product5/1
  Dot Product6/1 -> Add2/1
  Dot Product7/1 -> Add2/2
  Dot Product8/1 -> Add2/3
  Dot Product9/1 -> Add2/4
  a31/1 -> Dot Product6/1
  a32/1 -> Dot Product7/1
  a33/1 -> Dot Product8/1
  a35/1 -> Dot Product9/1
  a44/1 -> Dot Product10/1
  a55/1 -> Dot Product11/1
  a66/1 -> Dot Product12/1
  I1/1 -> Dot Product6/2, Dot Product3/2, Dot Product/2
  I2/1 -> Dot Product7/2, Dot Product4/2, Dot Product1/2
  I3/1 -> Dot Product8/2, Dot Product5/2, Dot Product2/2
  I4/1 -> Dot Product10/2
  I5/1 -> Dot Product9/2, Dot Product11/2
  I6/1 -> Dot Product12/2
  Add/1 -> A.I1/1
  Add1/1 -> A.I2/1
  Add2/1 -> A.I3/1
  Dot Product10/1 -> A.I4/1
  Dot Product11/1 -> A.I5/1
  Dot Product12/1 -> A.I6/1

== system PUMA_PID_dis/3-Link PUMA Robot-Block /secondLink ==
  ddteta2 : Inport
  Integrator : Integrator  LimitOutput=on  UpperSaturationLimit=10  LowerSaturationLimit=-10
  Integrator1 : Integrator  LimitOutput=on  UpperSaturationLimit=10  LowerSaturationLimit=-10
  Scope : Scope
  teta2 : Outport
  dteta2 : Outport  Port=2
  ddteta2. : Outport  Port=3
  wires:
  ddteta2/1 -> Scope/1, Integrator/1, ddteta2./1
  Integrator/1 -> Integrator1/1, dteta2/1
  Integrator1/1 -> teta2/1

== system PUMA_PID_dis/3-Link PUMA Robot-Block /thirdLink ==
  ddteta3 : Inport
  Integrator : Integrator  LimitOutput=on  UpperSaturationLimit=10  LowerSaturationLimit=-10
  Integrator1 : Integrator  LimitOutput=on  UpperSaturationLimit=10  LowerSaturationLimit=-10
  teta3 : Outport
  dteta3 : Outport  Port=2
  ddteta3. : Outport  Port=3
  wires:
  ddteta3/1 -> Integrator/1, ddteta3./1
  Integrator/1 -> Integrator1/1, dteta3/1
  Integrator1/1 -> teta3/1

== system PUMA_PID_dis/Fuzzy Controller/derivative ==
  teta1 : Inport
  teta2 : Inport  Port=2
  teta3 : Inport  Port=3
  desiredteta1 : Inport  Port=4
  desiredteta2 : Inport  Port=5
  desiredteta3 : Inport  Port=6
  Derivative{1..6} (6 alike) : Derivative  CoefficientInTFapproximation=0
  dteta1 : Outport
  dteta2 : Outport  Port=2
  dteta3 : Outport  Port=3
  desireddteta1 : Outport  Port=4
  desireddteta2 : Outport  Port=5
  desireddteta3 : Outport  Port=6
  wires:
  teta1/1 -> Derivative3/1
  teta2/1 -> Derivative1/1
  teta3/1 -> Derivative2/1
  desiredteta1/1 -> Derivative4/1
  desiredteta2/1 -> Derivative5/1
  desiredteta3/1 -> Derivative6/1
  Derivative3/1 -> dteta1/1
  Derivative1/1 -> dteta2/1
  Derivative2/1 -> dteta3/1
  Derivative4/1 -> desireddteta1/1
  Derivative5/1 -> desireddteta2/1
  Derivative6/1 -> desireddteta3/1

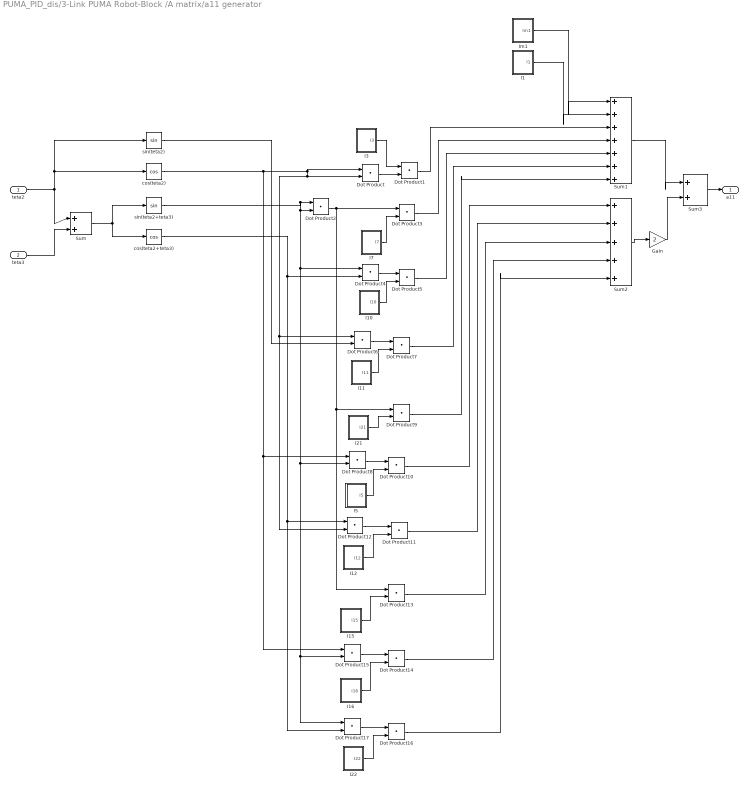
== system PUMA_PID_dis/3-Link PUMA Robot-Block /A matrix/a11 generator ==
  teta2 : Inport
  teta3 : Inport  Port=2
  Dot Product{,1..17} (18 alike) : DotProduct  InputSameDT=on  OutDataTypeStr=Inherit: Inherit via internal rule
  Gain : Gain  Gain=2
  I1 : Subsystem
  I10 : Subsystem
  I11 : Subsystem
  I12 : Subsystem
  I15 : Subsystem
  I16 : Subsystem
  I21 : Subsystem
  I22 : Subsystem
  I3 : Subsystem
  I5 : Subsystem
  I7 : Subsystem
  Im1 : Subsystem
  Sum : Sum  Inputs=|++
  Sum1 : Sum  Inputs=|+++++++
  Sum2 : Sum  Inputs=|+++++
  Sum3 : Sum  Inputs=|++
  cos(teta2) : Trigonometry  Operator=cos
  cos(teta2+teta3) : Trigonometry  Operator=cos
  sin(teta2) : Trigonometry
  sin(teta2+teta3) : Trigonometry
  a11 : Outport
  wires:
  teta2/1 -> Sum/1, cos(teta2)/1, sin(teta2)/1
  teta3/1 -> Sum/2
  Sum/1 -> sin(teta2+teta3)/1, cos(teta2+teta3)/1
  Sum2/1 -> Gain/1
  Sum1/1 -> Sum3/1
  Gain/1 -> Sum3/2
  Sum3/1 -> a11/1
  Im1/1(Im1) -> Sum1/1
  I1/1(I1) -> Sum1/2
  cos(teta2)/1 -> Dot Product/1, Dot Product/2, Dot Product6/1, Dot Product12/2, Dot Product8/1, Dot Product15/1
  I3/1(I3) -> Dot Product1/1
  Dot Product/1 -> Dot Product1/2
  Dot Product1/1 -> Sum1/3
  sin(teta2+teta3)/1 -> Dot Product2/1, Dot Product2/2, Dot Product4/1, Dot Product8/2, Dot Product15/2, Dot Product17/1
  Dot Product2/1 -> Dot Product3/1, Dot Product9/1, Dot Product13/1
  I7/1(I7) -> Dot Product3/2
  Dot Product3/1 -> Sum1/4
  Dot Product4/1 -> Dot Product5/1
  cos(teta2+teta3)/1 -> Dot Product4/2, Dot Product12/1, Dot Product17/2
  I10/1(I10) -> Dot Product5/2
  Dot Product5/1 -> Sum1/5
  sin(teta2)/1 -> Dot Product6/2
  Dot Product6/1 -> Dot Product7/1
  I11/1(I11) -> Dot Product7/2
  Dot Product7/1 -> Sum1/6
  I21/1(I21) -> Dot Product9/2
  Dot Product9/1 -> Sum1/7
  Dot Product8/1 -> Dot Product10/1
  I5/1(I5) -> Dot Product10/2
  Dot Product10/1 -> Sum2/1
  Dot Product12/1 -> Dot Product11/1
  I12/1(I12) -> Dot Product11/2
  Dot Product11/1 -> Sum2/2
  I15/1(I15) -> Dot Product13/2
  Dot Product13/1 -> Sum2/3
  Dot Product15/1 -> Dot Product14/1
  I16/1(I16) -> Dot Product14/2
  Dot Product14/1 -> Sum2/4
  Dot Product17/1 -> Dot Product16/1
  I22/1(I22) -> Dot Product16/2
  Dot Product16/1 -> Sum2/5

== system PUMA_PID_dis/3-Link PUMA Robot-Block /A matrix/a12 generator ==
  teta2 : Inport
  teta3 : Inport  Port=2
  Dot Product{,1..4} (5 alike) : DotProduct  InputSameDT=on  OutDataTypeStr=Inherit: Inherit via internal rule
  Gain : Gain  Gain=-1
  I13 : Subsystem
  I18 : Subsystem
  I4 : Subsystem
  I8 : Subsystem
  I9 : Subsystem
  Sum : Sum  Inputs=|++
  Sum3 : Sum  Inputs=|+++++
  cos(teta2) : Trigonometry  Operator=cos
  cos(teta2+teta3) : Trigonometry  Operator=cos
  sin(teta2) : Trigonometry
  sin(teta2+teta3) : Trigonometry
  a12 : Outport
  wires:
  teta2/1 -> sin(teta2)/1, cos(teta2)/1, Sum/1
  teta3/1 -> Sum/2
  Sum/1 -> sin(teta2+teta3)/1, cos(teta2+teta3)/1
  I4/1(I4) -> Dot Product/1
  sin(teta2)/1 -> Dot Product/2
  I8/1(I8) -> Dot Product1/1
  cos(teta2)/1 -> Dot Product2/1
  I9/1(I9) -> Dot Product2/2
  cos(teta2+teta3)/1 -> Dot Product1/2, Dot Product4/1
  I13/1(I13) -> Dot Product3/2
  sin(teta2+teta3)/1 -> Dot Product3/1
  I18/1(I18) -> Dot Product4/2
  Dot Product4/1 -> Gain/1
  Sum3/1 -> a12/1
  Dot Product/1 -> Sum3/1
  Dot Product2/1 -> Sum3/2
  Dot Product1/1 -> Sum3/3
  Dot Product3/1 -> Sum3/4
  Gain/1 -> Sum3/5

== system PUMA_PID_dis/3-Link PUMA Robot-Block /A matrix/a13 generator ==
  teta2 : Inport
  teta3 : Inport  Port=2
  Dot Product1 : DotProduct  InputSameDT=on  OutDataTypeStr=Inherit: Inherit via internal rule
  Dot Product3 : DotProduct  InputSameDT=on  OutDataTypeStr=Inherit: Inherit via internal rule
  Dot Product4 : DotProduct  InputSameDT=on  OutDataTypeStr=Inherit: Inherit via internal rule
  Gain : Gain  Gain=-1
  I13 : Subsystem
  I18 : Subsystem
  I8 : Subsystem
  Sum : Sum  Inputs=|++
  Sum3 : Sum  Inputs=|+++
  cos(teta2+teta3) : Trigonometry  Operator=cos
  sin(teta2+teta3) : Trigonometry
  a13 : Outport
  wires:
  teta2/1 -> Sum/1
  teta3/1 -> Sum/2
  Sum/1 -> sin(teta2+teta3)/1, cos(teta2+teta3)/1
  I8/1(I8) -> Dot Product1/1
  cos(teta2+teta3)/1 -> Dot Product1/2, Dot Product4/1
  I13/1(I13) -> Dot Product3/2
  sin(teta2+teta3)/1 -> Dot Product3/1
  I18/1(I18) -> Dot Product4/2
  Dot Product4/1 -> Gain/1
  Sum3/1 -> a13/1
  Dot Product1/1 -> Sum3/1
  Dot Product3/1 -> Sum3/2
  Gain/1 -> Sum3/3

== system PUMA_PID_dis/3-Link PUMA Robot-Block /A matrix/a22 generator ==
  teta2 : Inport
  teta3 : Inport  Port=2
  Dot Product1 : DotProduct  InputSameDT=on  OutDataTypeStr=Inherit: Inherit via internal rule
  Dot Product2 : DotProduct  InputSameDT=on  OutDataTypeStr=Inherit: Inherit via internal rule
  Dot Product4 : DotProduct  InputSameDT=on  OutDataTypeStr=Inherit: Inherit via internal rule
  Gain : Gain  Gain=2
  I12 : Subsystem
  I15 : Subsystem
  I16 : Subsystem
  I2 : Subsystem
  I5 : Subsystem
  I6 : Subsystem
  Im2 : Subsystem
  Sum1 : Sum  Inputs=|++++
  Sum3 : Sum  Inputs=|++++
  cos(teta2) : Trigonometry  Operator=cos
  sin(teta3) : Trigonometry
  a22 : Outport
  wires:
  teta2/1 -> cos(teta2)/1
  teta3/1 -> sin(teta3)/1
  Sum3/1 -> a22/1
  Im2/1(Im2) -> Sum3/1
  I2/1(I2) -> Sum3/2
  I6/1(I6) -> Sum3/3
  Gain/1 -> Sum3/4
  sin(teta3)/1 -> Dot Product4/1, Dot Product2/1
  I5/1(I5) -> Dot Product4/2
  I12/1(I12) -> Dot Product1/2
  cos(teta2)/1 -> Dot Product1/1
  I16/1(I16) -> Dot Product2/2
  Sum1/1 -> Gain/1
  I15/1(I15) -> Sum1/1
  Dot Product1/1 -> Sum1/2
  Dot Product4/1 -> Sum1/3
  Dot Product2/1 -> Sum1/4

== system PUMA_PID_dis/3-Link PUMA Robot-Block /A matrix/a23 generator ==
  teta3 : Inport
  Dot Product1 : DotProduct  InputSameDT=on  OutDataTypeStr=Inherit: Inherit via internal rule
  Dot Product2 : DotProduct  InputSameDT=on  OutDataTypeStr=Inherit: Inherit via internal rule
  Dot Product4 : DotProduct  InputSameDT=on  OutDataTypeStr=Inherit: Inherit via internal rule
  Gain : Gain  Gain=2
  I12 : Subsystem
  I15 : Subsystem
  I16 : Subsystem
  I5 : Subsystem
  I6 : Subsystem
  Sum3 : Sum  Inputs=|+++++
  cos(teta3) : Trigonometry  Operator=cos
  sin(teta3) : Trigonometry
  a23 : Outport
  wires:
  teta3/1 -> sin(teta3)/1, cos(teta3)/1
  Sum3/1 -> a23/1
  sin(teta3)/1 -> Dot Product4/1, Dot Product2/1
  I5/1(I5) -> Dot Product4/2
  I12/1(I12) -> Dot Product1/1
  cos(teta3)/1 -> Dot Product1/2
  I16/1(I16) -> Dot Product2/2
  I15/1(I15) -> Gain/1
  Gain/1 -> Sum3/1
  Dot Product1/1 -> Sum3/2
  I6/1(I6) -> Sum3/3
  Dot Product4/1 -> Sum3/4
  Dot Product2/1 -> Sum3/5

== system PUMA_PID_dis/3-Link PUMA Robot-Block /A matrix/a33 generator ==
  Gain : Gain  Gain=2
  I15 : Subsystem
  I6 : Subsystem
  Im3 : Subsystem
  Sum3 : Sum  Inputs=|+++
  a33 : Outport
  wires:
  Sum3/1 -> a33/1
  I15/1(I15) -> Gain/1
  Gain/1 -> Sum3/1
  I6/1(I6) -> Sum3/2
  Im3/1(Im3) -> Sum3/3

== system PUMA_PID_dis/3-Link PUMA Robot-Block /A matrix/a35 generator ==
  I15 : Subsystem
  I17 : Subsystem
  Sum3 : Sum  Inputs=|++
  a35 : Outport
  wires:
  Sum3/1 -> a35/1
  I15/1(I15) -> Sum3/1
  I17/1(I17) -> Sum3/2

== system PUMA_PID_dis/3-Link PUMA Robot-Block /A matrix/a44 generator ==
  I14 : Subsystem
  Im4 : Subsystem
  Sum3 : Sum  Inputs=|++
  a44 : Outport
  wires:
  Sum3/1 -> a44/1
  Im4/1(Im4) -> Sum3/1
  I14/1(I14) -> Sum3/2

== system PUMA_PID_dis/3-Link PUMA Robot-Block /A matrix/a55 generator ==
  I17 : Subsystem
  Im5 : Subsystem
  Sum3 : Sum  Inputs=|++
  a55 : Outport
  wires:
  Sum3/1 -> a55/1
  Im5/1(Im5) -> Sum3/1
  I17/1(I17) -> Sum3/2

== system PUMA_PID_dis/3-Link PUMA Robot-Block /A matrix/a66 generator ==
  I23 : Subsystem
  Im6 : Subsystem
  Sum3 : Sum  Inputs=|++
  a66 : Outport
  wires:
  Sum3/1 -> a66/1
  Im6/1(Im6) -> Sum3/1
  I23/1(I23) -> Sum3/2

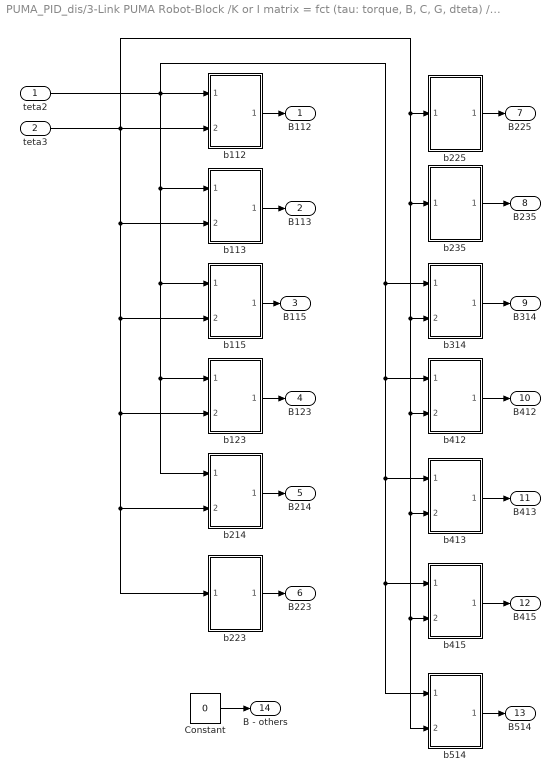
== system PUMA_PID_dis/3-Link PUMA Robot-Block /K or I matrix = fct (tau: torque, B, C, G, dteta) /B matrix ==
  teta2 : Inport
  teta3 : Inport  Port=2
  Constant : Constant  Value=0
  b112 : Subsystem
  b113 : Subsystem
  b115 : Subsystem
  b123 : Subsystem
  b214 : Subsystem
  b223 : Subsystem
  b225 : Subsystem
  b235 : Subsystem
  b314 : Subsystem
  b412 : Subsystem
  b413 : Subsystem
  b415 : Subsystem
  b514 : Subsystem
  B112 : Outport
  B113 : Outport  Port=2
  B115 : Outport  Port=3
  B123 : Outport  Port=4
  B214 : Outport  Port=5
  B223 : Outport  Port=6
  B225 : Outport  Port=7
  B235 : Outport  Port=8
  B314 : Outport  Port=9
  B412 : Outport  Port=10
  B413 : Outport  Port=11
  B415 : Outport  Port=12
  B514 : Outport  Port=13
  B - others : Outport  Port=14
  wires:
  b112/1(b112) -> B112/1
  b113/1(b113) -> B113/1
  b115/1(b115) -> B115/1
  b123/1(b123) -> B123/1
  b214/1(b214) -> B214/1
  b223/1(b223) -> B223/1
  b225/1(b225) -> B225/1
  b235/1(b235) -> B235/1
  b314/1(b314) -> B314/1
  b412/1(b412) -> B412/1
  b413/1(b413) -> B413/1
  b415/1(b415) -> B415/1
  b514/1(b514) -> B514/1
  teta2/1 -> b514/1(teta2), b415/1(teta2), b413/1(teta2), b412/1(teta2), b314/1(teta2), b214/1(teta2), b123/1(teta2), b115/1(teta2), b113/1(teta2), b112/1(teta2)
  teta3/1 -> b514/2(teta3), b415/2(teta3), b413/2(teta3), b412/2(teta3), b314/2(teta3), b235/1(teta3), b225/1(teta3), b223/1(teta3), b214/2(teta3), b123/2(teta3), b115/2(teta3), b113/2(teta3), b112/2(teta3)
  Constant/1 -> B - others/1

== system PUMA_PID_dis/3-Link PUMA Robot-Block /K or I matrix = fct (tau: torque, B, C, G, dteta) /C matrix ==
  teta3 : Inport
  teta2 : Inport  Port=2
  Constant : Constant  Value=0
  c12 : Subsystem
  c13 : Subsystem
  c21 : Subsystem
  c23 : Subsystem
  c31 : Subsystem
  c32 : Subsystem
  c51 : Subsystem
  c52 : Subsystem
  C12 : Outport
  C13 : Outport  Port=2
  C52 : Outport  Port=3
  C21 : Outport  Port=4
  C23 : Outport  Port=5
  C31 : Outport  Port=6
  C32 : Outport  Port=7
  C51 : Outport  Port=8
  C-others : Outport  Port=9
  wires:
  c12/1(c12) -> C12/1
  c13/1(c13) -> C13/1
  c21/1(c21) -> C21/1
  c23/1(c23) -> C23/1
  c31/1(c31) -> C31/1
  c32/1(c32) -> C32/1
  c51/1(c51) -> C51/1
  c52/1(c52) -> C52/1
  Constant/1 -> C-others/1
  teta3/1 -> c52/1(teta3), c51/2(teta3), c32/1(teta3), c31/2(teta3), c23/1(teta3), c21/2(teta3), c13/2(teta3), c12/1(teta3)
  teta2/1 -> c13/1(teta2), c51/1(teta2), c31/1(teta2), c21/1(teta2), c12/2(teta2)

== system PUMA_PID_dis/3-Link PUMA Robot-Block /K or I matrix = fct (tau: torque, B, C, G, dteta) /Gravity matrix ==
  teta2 : Inport
  teta3 : Inport  Port=2
  Constant : Constant  Value=0
  g2 term : Subsystem
  g3 term : Subsystem
  g5 term : Subsystem
  g1 : Outport
  g2 : Outport  Port=2
  g3 : Outport  Port=3
  g4 : Outport  Port=4
  g5 : Outport  Port=5
  g6 : Outport  Port=6
  wires:
  teta2/1 -> g5 term/1(teta2), g3 term/1(teta2), g2 term/1(teta2)
  teta3/1 -> g5 term/2(teta3), g3 term/2(teta3), g2 term/2(teta3)
  Constant/1 -> g1/1, g4/1, g6/1
  g2 term/1(G2) -> g2/1
  g3 term/1(G3) -> g3/1
  g5 term/1(G5) -> g5/1

== system PUMA_PID_dis/3-Link PUMA Robot-Block /A matrix/a11 generator/I1 ==
  AI1 actual I1 : Constant  Value=1.43
  Sum4 : Sum  Inputs=|++
  UI1 uncertainty added to I1 +- 0.27 max : Constant  Value=UI1
  I1 : Outport
  wires:
  AI1 actual I1/1 -> Sum4/1
  UI1 uncertainty added to I1 +- 0.27 max/1 -> Sum4/2
  Sum4/1 -> I1/1

== system PUMA_PID_dis/3-Link PUMA Robot-Block /A matrix/a11 generator/I10 ==
  AI10 actual I10 : Constant  Value=-0.0213
  Sum4 : Sum  Inputs=|++
  UI10 uncertainty added to I10 +- 0.022 max : Constant  Value=UI10
  I10 : Outport
  wires:
  AI10 actual I10/1 -> Sum4/1
  UI10 uncertainty added to I10 +- 0.022 max/1 -> Sum4/2
  Sum4/1 -> I10/1

== system PUMA_PID_dis/3-Link PUMA Robot-Block /A matrix/a11 generator/I11 ==
  AI11 actual I11 : Constant  Value=-0.0142
  Sum4 : Sum  Inputs=|++
  UI11 uncertainty added to I11 +- 0.007 max : Constant  Value=UI11
  I11 : Outport
  wires:
  AI11 actual I11/1 -> Sum4/1
  UI11 uncertainty added to I11 +- 0.007 max/1 -> Sum4/2
  Sum4/1 -> I11/1

== system PUMA_PID_dis/3-Link PUMA Robot-Block /A matrix/a11 generator/I12 ==
  AI12 actual I12 : Constant  Value=-0.011
  Sum4 : Sum  Inputs=|++
  UI12 uncertainty added to I12 +- 0.0011 max : Constant  Value=UI12
  I12 : Outport
  wires:
  AI12 actual I12/1 -> Sum4/1
  UI12 uncertainty added to I12 +- 0.0011 max/1 -> Sum4/2
  Sum4/1 -> I12/1

== system PUMA_PID_dis/3-Link PUMA Robot-Block /A matrix/a11 generator/I15 ==
  AI15 actual I15 : Constant  Value=0.00125
  Sum4 : Sum  Inputs=|++
  UI15 uncertainty added to I15 +- 0.0003 max : Constant  Value=UI15
  I15 : Outport
  wires:
  AI15 actual I15/1 -> Sum4/1
  UI15 uncertainty added to I15 +- 0.0003 max/1 -> Sum4/2
  Sum4/1 -> I15/1

== system PUMA_PID_dis/3-Link PUMA Robot-Block /A matrix/a11 generator/I16 ==
  AI16 actual I16 : Constant  Value=0.00124
  Sum4 : Sum  Inputs=|++
  UI16 uncertainty added to I16 +- 0.0003 max : Constant  Value=UI16
  I16 : Outport
  wires:
  AI16 actual I16/1 -> Sum4/1
  UI16 uncertainty added to I16 +- 0.0003 max/1 -> Sum4/2
  Sum4/1 -> I16/1

== system PUMA_PID_dis/3-Link PUMA Robot-Block /A matrix/a11 generator/I21 ==
  AI21 actual I21 : Constant  Value=-0.0001
  Sum4 : Sum  Inputs=|++
  UI21 uncertainty added to I21 +- 0.0006 max : Constant  Value=UI21
  I21 : Outport
  wires:
  AI21 actual I21/1 -> Sum4/1
  UI21 uncertainty added to I21 +- 0.0006 max/1 -> Sum4/2
  Sum4/1 -> I21/1

== system PUMA_PID_dis/3-Link PUMA Robot-Block /A matrix/a11 generator/I22 ==
  AI22 actual I22 : Constant  Value=-0.000058
  Sum4 : Sum  Inputs=|++
  UI22 uncertainty added to I22 +- 0.000015 max : Constant  Value=UI22
  I22 : Outport
  wires:
  AI22 actual I22/1 -> Sum4/1
  UI22 uncertainty added to I22 +- 0.000015 max/1 -> Sum4/2
  Sum4/1 -> I22/1

== system PUMA_PID_dis/3-Link PUMA Robot-Block /A matrix/a11 generator/I3 ==
  AI3 actual I3 : Constant  Value=1.38
  Sum4 : Sum  Inputs=|++
  UI3 uncertainty added to I3 +- 0.05 max : Constant  Value=UI3
  I3 : Outport
  wires:
  AI3 actual I3/1 -> Sum4/1
  UI3 uncertainty added to I3 +- 0.05 max/1 -> Sum4/2
  Sum4/1 -> I3/1

== system PUMA_PID_dis/3-Link PUMA Robot-Block /A matrix/a11 generator/I5 ==
  AI5 actual I5 : Constant  Value=0.372
  Sum4 : Sum  Inputs=|++
  UI5 uncertainty added to I5 +- 0.05 max : Constant  Value=UI5
  I5 : Outport
  wires:
  AI5 actual I5/1 -> Sum4/1
  UI5 uncertainty added to I5 +- 0.05 max/1 -> Sum4/2
  Sum4/1 -> I5/1

== system PUMA_PID_dis/3-Link PUMA Robot-Block /A matrix/a11 generator/I7 ==
  AI7 actual I7 : Constant  Value=0.298
  Sum4 : Sum  Inputs=|++
  UI7 uncertainty added to I7 +- 0.029 max : Constant  Value=UI7
  I7 : Outport
  wires:
  AI7 actual I7/1 -> Sum4/1
  UI7 uncertainty added to I7 +- 0.029 max/1 -> Sum4/2
  Sum4/1 -> I7/1

== system PUMA_PID_dis/3-Link PUMA Robot-Block /A matrix/a11 generator/Im1 ==
  AIm1 actual Im1 : Constant  Value=1.14
  Sum4 : Sum  Inputs=|++
  UIm1 uncertainty added to Im1 +- 0.27 max : Constant  Value=UIm1
  Im1 : Outport
  wires:
  AIm1 actual Im1/1 -> Sum4/1
  UIm1 uncertainty added to Im1 +- 0.27 max/1 -> Sum4/2
  Sum4/1 -> Im1/1

== system PUMA_PID_dis/3-Link PUMA Robot-Block /A matrix/a12 generator/I13 ==
  AI13 actual I13 : Constant  Value=-0.00379
  Sum4 : Sum  Inputs=|++
  UI13 uncertainty added to I13 +- 0.0009 max : Constant  Value=UI13
  I13 : Outport
  wires:
  AI13 actual I13/1 -> Sum4/1
  UI13 uncertainty added to I13 +- 0.0009 max/1 -> Sum4/2
  Sum4/1 -> I13/1

== system PUMA_PID_dis/3-Link PUMA Robot-Block /A matrix/a12 generator/I18 ==
  AI18 actual I18 : Constant  Value=0.000431
  Sum4 : Sum  Inputs=|++
  UI18 uncertainty added to I18 +- 0.0003 max : Constant  Value=UI18
  I18 : Outport
  wires:
  AI18 actual I18/1 -> Sum4/1
  UI18 uncertainty added to I18 +- 0.0003 max/1 -> Sum4/2
  Sum4/1 -> I18/1

== system PUMA_PID_dis/3-Link PUMA Robot-Block /A matrix/a12 generator/I4 ==
  AI4 actual I4 : Constant  Value=0.69
  Sum4 : Sum  Inputs=|++
  UI4 uncertainty added to I4 +- 0.02 max : Constant  Value=UI4
  I4 : Outport
  wires:
  AI4 actual I4/1 -> Sum4/1
  UI4 uncertainty added to I4 +- 0.02 max/1 -> Sum4/2
  Sum4/1 -> I4/1
